simulink model "liti4_7xiti"  (Simulink 5.0)
settings: Solver=ode45  SolverMode=SingleTasking  StartTime=0.0  StopTime=3  FixedStep=0.1  RelTol=1e-3
libraries: cstblocks x2
settings Model: LastModifiedBy=Administrator

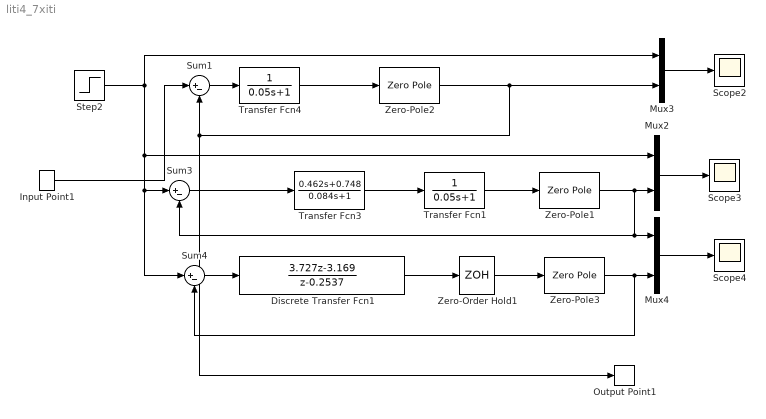
== system liti4_7xiti ==
  Discrete Transfer Fcn1 : DiscreteTransferFcn  Numerator=[3.727 -3.169]  Denominator=[1 -0.2537]  SampleTime=0.1
  Input Point1 : cstblocks/Input Point
  Mux2 : Mux  Inputs=2
  Mux3 : Mux  Inputs=2
  Mux4 : Mux  Inputs=2
  Output Point1 : cstblocks/Output Point
  Scope2 : Scope
      settings: YMin=-3.5  YMax=1  MaxDataPoints=500000
  Scope3 : Scope
      settings: YMin=-3.5  YMax=1  SaveName=ScopeData2  MaxDataPoints=500000
  Scope4 : Scope
      settings: YMin=-3.5  YMax=1  SaveName=yyy  DataFormat=Array  MaxDataPoints=500000
  Step2 : Step  Time=0  SampleTime=0
  Sum1 : Sum  Inputs=|+-  SaturateOnIntegerOverflow=on
  Sum3 : Sum  Inputs=|+-  SaturateOnIntegerOverflow=on
  Sum4 : Sum  Inputs=|+-  SaturateOnIntegerOverflow=on
  Transfer Fcn1 : TransferFcn  Denominator=[0.05 1]
  Transfer Fcn3 : TransferFcn  Numerator=[0.462 0.748]  Denominator=[0.084 1]
  Transfer Fcn4 : TransferFcn  Denominator=[0.05 1]
  Zero-Order Hold1 : ZeroOrderHold  SampleTime=0.1
  Zero-Pole1 : ZeroPole  Zeros=[]  Poles=[0 -1]  Gain=[10]
  Zero-Pole2 : ZeroPole  Zeros=[]  Poles=[0 -1]  Gain=[10]
  Zero-Pole3 : ZeroPole  Zeros=[]  Poles=[0 -1]  Gain=[10]
  wires:
  Step2/1 -> Mux2/1, Sum3/1, Sum4/1, Mux3/1
  Mux2/1 -> Scope3/1
  Zero-Pole1/1 -> Mux2/2, Mux4/1, Sum3/2
  Mux3/1 -> Scope2/1
  Zero-Pole2/1 -> Mux3/2, Sum1/2, Output Point1/1
  Sum1/1 -> Transfer Fcn4/1
  Sum3/1 -> Transfer Fcn3/1
  Mux4/1 -> Scope4/1
  Zero-Pole3/1 -> Mux4/2, Sum4/2
  Discrete Transfer Fcn1/1 -> Zero-Order Hold1/1
  Sum4/1 -> Discrete Transfer Fcn1/1
  Zero-Order Hold1/1 -> Zero-Pole3/1
  Transfer Fcn3/1 -> Transfer Fcn1/1
  Transfer Fcn4/1 -> Zero-Pole2/1
  Transfer Fcn1/1 -> Zero-Pole1/1
  Input Point1/1 -> Sum1/1
